simulink model "minmax_multi_test"  (Simulink 7.2)
settings: Solver=ode45  StartTime=0.0  StopTime=10.0  RelTol=1e-3
settings Model: Creator=arnaud  LastModifiedBy=arnaud
settings DataIOCC: SaveFormat=Structure

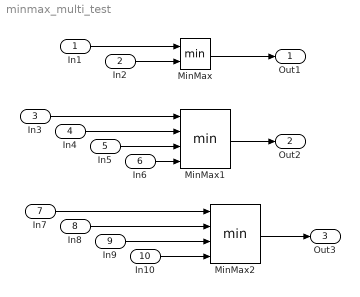
== system minmax_multi_test ==
  In1 : Inport  PortDimensions=1  OutDataType=sfix(16)  OutScaling=2^0
  In2 : Inport  Port=2  PortDimensions=5  OutDataType=sfix(16)  OutScaling=2^0
  In3 : Inport  Port=3  PortDimensions=1  OutDataType=sfix(16)  OutScaling=2^0
  In4 : Inport  Port=4  PortDimensions=3  OutDataType=sfix(16)  OutScaling=2^0
  In5 : Inport  Port=5  PortDimensions=3  OutDataType=sfix(16)  OutScaling=2^0
  In6 : Inport  Port=6  PortDimensions=3  OutDataType=sfix(16)  OutScaling=2^0
  In7 : Inport  Port=7  PortDimensions=1  OutDataType=sfix(16)  OutScaling=2^0
  In8 : Inport  Port=8  PortDimensions=1  OutDataType=sfix(16)  OutScaling=2^0
  In9 : Inport  Port=9  PortDimensions=[2 3]  OutDataType=sfix(16)  OutScaling=2^0
  In10 : Inport  Port=10  PortDimensions=[2 3]  OutDataType=sfix(16)  OutScaling=2^0
  MinMax : MinMax  Inputs=2  OutDataType=sfix(16)  OutScaling=2^0
  MinMax1 : MinMax  Inputs=4  OutDataType=sfix(16)  OutScaling=2^0
  MinMax2 : MinMax  Inputs=4  OutDataType=sfix(16)  OutScaling=2^0
  Out1 : Outport  OutDataType=sfix(16)  OutScaling=2^0
  Out2 : Outport  Port=2  OutDataType=sfix(16)  OutScaling=2^0
  Out3 : Outport  Port=3  OutDataType=sfix(16)  OutScaling=2^0
  wires:
  MinMax/1 -> Out1/1
  In1/1 -> MinMax/1
  In2/1 -> MinMax/2
  MinMax1/1 -> Out2/1
  In3/1 -> MinMax1/1
  In4/1 -> MinMax1/2
  In5/1 -> MinMax1/3
  In6/1 -> MinMax1/4
  MinMax2/1 -> Out3/1
  In7/1 -> MinMax2/1
  In8/1 -> MinMax2/2
  In9/1 -> MinMax2/3
  In10/1 -> MinMax2/4
